simulink model "3Dsimulation"  (R2021b)
settings: Solver=VariableStepAuto  StartTime=0.0  StopTime=10.5  RelTol=1e-3
libraries: sim3dcameralib x1, sim3dlib x1, sim3dautolib x1, dspvision x1
settings Model: Creator=The MathWorks, Inc.  LastModifiedBy=大亲亲子
settings SolverCC: AlgebraicLoopSolver=TrustRegion
settings DebuggingCC: SFMachineParentedDataDiag=warning

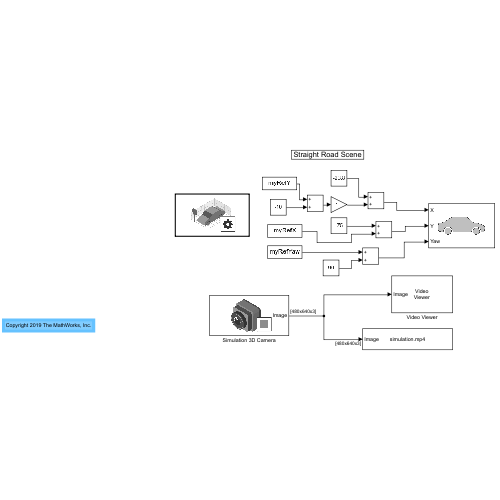
[thumbnail: Simulink's stored preview of the top-level diagram]
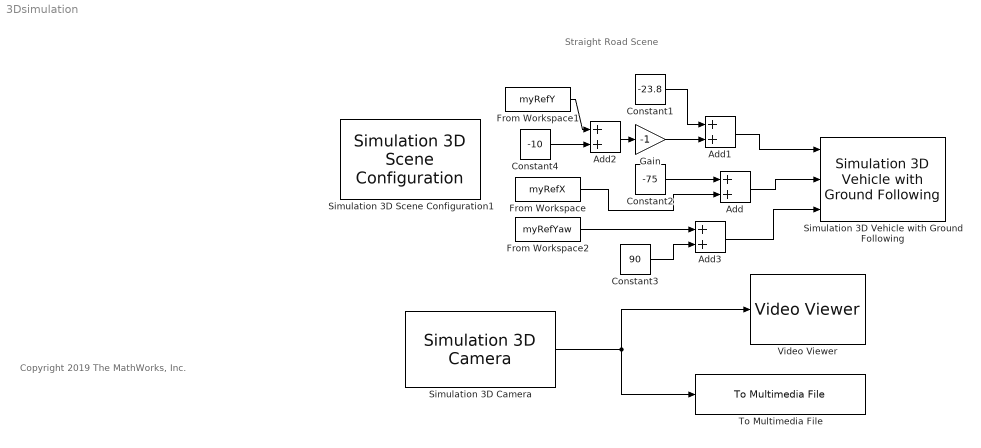
== system 3Dsimulation ==
  note: Straight Road Scene
  note: Copyright 2019 The MathWorks, Inc.
  Add{,1..3} (4 alike) : Sum
  Constant1 : Constant  Value=-23.8
  Constant2 : Constant  Value=-75
  Constant3 : Constant  Value=90
  Constant4 : Constant  Value=-10
  From Workspace : FromWorkspace  VariableName=myRefX  OutDataTypeStr=double  SampleTime=0.05
  From Workspace1 : FromWorkspace  VariableName=myRefY  OutDataTypeStr=double  SampleTime=0.05
  From Workspace2 : FromWorkspace  VariableName=myRefYaw  OutDataTypeStr=double  SampleTime=0.05
  Gain : Gain  Gain=-1
  Simulation 3D Camera : sim3dcameralib/Simulation 3D Camera  sensorTag=Sim3dSensor1  sensorId=1  sensorName=Sim3dSensor1  vehTagList={'Scene Origin';'SimulinkVehicle1'}  vehTag=SimulinkVehicle1  mountLoc=Roof center  offsetFlag=off  tmountOffset=[0, 0, 0]  extTmount=off  rmountOffset=[0, 0, 0]  extRmount=off  FocalLength=[320, 320]  OpticalCenter=[640, 480]/2  ImageSize=[480, 640]  RadialDistortion=[0, 0]  TangentialDistortion=[0, 0]  SensorSkew=0  DepthOutportEnabled=off  SemanticOutportEnabled=off  TransformOutportEnabled=off  SampleTime=-1  mountPoint=[-0.560000002384186 0 1.99000000953674]  mountOrientation=[0 0 0]  aMode=3  ID=1
      settings: SourceProductBaseCode=AE,DR,UV,VE
  Simulation 3D Scene Configuration1 : sim3dlib/Simulation 3D Scene Configuration  Priority=0  ProjectFormat_internal=Unreal Editor  ProjectFormat=Unreal Editor  SceneDesc=Straight road  ProjectName=F:\Program Files\MATLAB\R2021b\toolbox\shared\sim3d_projects\automotive_project\UE4\WindowsNoEditor\VehicleSimulation.exe  ScenePath=/Game/Maps/HwStrght  UEProjPath=F:\Local\AutoVrtlEnv\AutoVrtlEnv.uproject  vehTagList={'Scene Origin';'SimulinkVehicle1'}  vehTag=SimulinkVehicle1  OpVisEn=off  Ts=1/60  EnableWindow=on  EnableWeather=off  SunAltitude=40.0  SunAzimuth=90  clouds=10  wind=1  fog=0  rain=0  sensorTag=MainCamera2  sensorId=2  sensorName=MainCamera2  mountLoc=Origin  offsetFlag=off  tmountOffset=[0, 0, 0]  rmountOffset=[0, 0, 0]  HorizontalResolution=1280  VerticalResolution=720  HorizontalFOV=60  mountPoint=[0 0 0]  mountOrientation=[0 0 0]  aMode=3  ID=2
      settings: SourceProductBaseCode=AE,DR,UV,VE
  Simulation 3D Vehicle with Ground Following : sim3dautolib/Simulation 3D Vehicle with Ground Following  Priority=-1  PassVehMesh=Sport utility vehicle  PassVehMesh_Internal=Sport utility vehicle  MeshPath=/MathWorksSimulation/Vehicles/Muscle/Meshes/SK_MuscleCar.SK_MuscleCar  TrackWidth=1.9  WheelBase=3  WheelRadius=0.35  VehColor=Red  VehColor_Internal=Red  InitialPos=[1, 0, 0]  InitialRot=[0, 0, 0]  ActorName=SimulinkVehicle1  SampleTime=-1  ActorType=SimulinkVehicle  ID=1  aMode=3  ActorTag=SimulinkVehicle1  CoordinateScheme=ISO  VehLightsControl=off  HeadlightColor=[ 1, 1, 1 ]  HighBeamIntensity=100000  LowBeamIntensity=60000  HighBeamConeAngle=70  LowBeamConeAngle=70  LeftHeadlightOrientation=[ 0, 0 ]  RightHeadlightOrientation=[ 0, 0 ]  BrakelightIntensity=500  ReverselightIntensity=500  SignallightIntensity=500  SignallightPeriod=1  SignalPulseWidth=50  TransformOutportEnabled=off
      settings: SourceProductBaseCode=AE,DR,UV,VE
  To Multimedia File : dspvision/To Multimedia File  outputFilename=simulation.mp4  streamSelection=Video only  videoCompressor=None (uncompressed)  audioCompressor=None (uncompressed)  imagePorts=One multidimensional signal  fileType=MPEG4  audioDatatype=Determine from input data type  fourcc=RGB  videoQuality=100  mj2000CompFactor=10
  Video Viewer : VideoViewer  FigPos=[553 740.4 680 522.4]
  wires:
  Add1/1 -> Simulation 3D Vehicle with Ground Following/1
  Add/1 -> Simulation 3D Vehicle with Ground Following/2
  Constant1/1 -> Add1/1
  Constant2/1 -> Add/1
  From Workspace/1 -> Add/2
  From Workspace1/1 -> Add2/1
  Constant4/1 -> Add2/2
  Gain/1 -> Add1/2
  Add2/1 -> Gain/1
  From Workspace2/1 -> Add3/1
  Constant3/1 -> Add3/2
  Add3/1 -> Simulation 3D Vehicle with Ground Following/3
  Simulation 3D Camera/1 -> To Multimedia File/1, Video Viewer/1
